simulink model "powertrain"  (R2020b)
settings: Solver=FixedStepAuto  StartTime=0.0  StopTime=t(end)  RelTol=1e-3
PreLoadFcn:
  | C_sc = 1;
StartFcn:
  | C_sc = 1;
values from neighbouring files (symbols this model uses):
  D = 0    [model_fc.m]
  Ts = old_data.Ts    [model_fc.m]
undefined symbols (not defined in the file or in its folder): ANFIS, command, DiscIntNeverNeededParam, ECMS, Flight, in, Ion, Lithium, MPC, out, Tmpc, w
libraries: powerlib x25, neural x25, fuzblock x5, electricdrivelib x3, lib_converters x3, simulink x3, re_lib x1
(part 3 of 8)

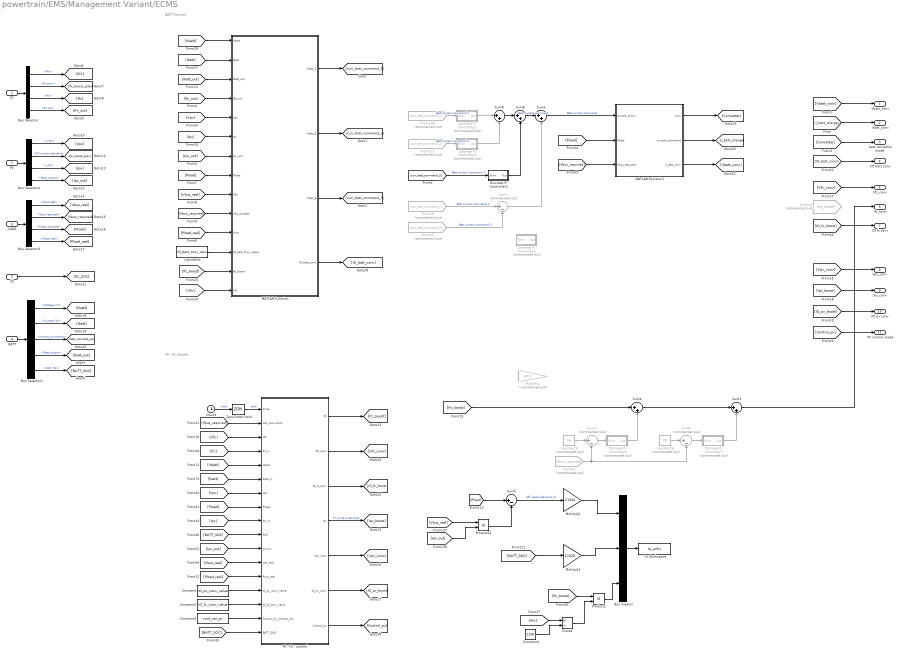
== system powertrain/EMS/Management Variant/ECMS ==
  note: PV - FC Control
  note: BATT Control
  PV : Inport
  FC : Inport  Port=2
  SC : Inport  Port=3
  BATT : Inport  Port=4
  LOAD : Inport  Port=5
  Bus Creator : BusCreator  Inputs=3
  Bus Selector : BusSelector  OutputSignals=Vfc,Ifc conv,Ifc,Ifc out
  Bus Selector1 : BusSelector  OutputSignals=Voltage (V),Current (A),current_command,Ibatt_output,SOC (%)
  Bus Selector2 : BusSelector  OutputSignals=V_PV,PV current demand,I_PV,Ibatt_output
  Bus Selector3 : BusSelector  OutputSignals=Vbus real,Vbus required,Pload required,Pload real
  Clock3 : Clock
  Constant : Constant  Value=IO_pv_conv_value
  Constant1 : Constant  Value=1100
  Constant2 : Constant  Value=IO_fc_conv_value
  Constant3 : Constant  Value=cont_var_pv
  Constant4 : Constant  Value=IO_batt_conv_value
  Constant5 : Constant  Commented=on  Value=74
  Constant6 : Constant  Commented=on  Value=70
  Discrete PI Controller1 : Subsystem  Commented=on  DialogController=POWERSYS.PowerSysDialog  mask(Discrete PI Controller){Kp=1, Ki=10, Par_Limits=[100 -100], Init=0, Ts=1e-4}
      mask prompts: Kp "Proportional gain (Kp):"; Ki "Integral gain (Ki):"; Par_Limits "Output limits: [ Upper   Lower ]"; Init "Output initial value:"; Ts "Sample time:"
      mask help: This block implements a discrete PI controller.
      mask init:
      | UpperLimit=Par_Limits(1);
      | LowerLimit=Par_Limits(2);
      | power_initmask();
      mask Help: This block is part of a subset of blocks in the Extras library that does not have documentation associated with it, other than the block mask description.
      mask Display: disp('PI');
  Discrete PI Controller2 : Subsystem  DialogController=POWERSYS.PowerSysDialog  mask(Discrete PI Controller){Kp=10, Ki=100, Par_Limits=[30 -4], Init=0, Ts=Ts}
      mask prompts: Kp "Proportional gain (Kp):"; Ki "Integral gain (Ki):"; Par_Limits "Output limits: [ Upper   Lower ]"; Init "Output initial value:"; Ts "Sample time:"
      mask help: This block implements a discrete PI controller.
      mask init:
      | UpperLimit=Par_Limits(1);
      | LowerLimit=Par_Limits(2);
      | power_initmask();
      mask Help: This block is part of a subset of blocks in the Extras library that does not have documentation associated with it, other than the block mask description.
      mask Display: disp('PI');
  Discrete PI Controller3 : Subsystem  Commented=on  DialogController=POWERSYS.PowerSysDialog  mask(Discrete PI Controller){Kp=10, Ki=1, Par_Limits=[100 -100], Init=0, Ts=1e-4}
      mask prompts: Kp "Proportional gain (Kp):"; Ki "Integral gain (Ki):"; Par_Limits "Output limits: [ Upper   Lower ]"; Init "Output initial value:"; Ts "Sample time:"
      mask help: This block implements a discrete PI controller.
      mask init:
      | UpperLimit=Par_Limits(1);
      | LowerLimit=Par_Limits(2);
      | power_initmask();
      mask Help: This block is part of a subset of blocks in the Extras library that does not have documentation associated with it, other than the block mask description.
      mask Display: disp('PI');
  Discrete PI Controller5 : Subsystem  Commented=on  DialogController=POWERSYS.PowerSysDialog  mask(Discrete PI Controller){Kp=10, Ki=10, Par_Limits=[50 -20], Init=0, Ts=1e-4}
      mask prompts: Kp "Proportional gain (Kp):"; Ki "Integral gain (Ki):"; Par_Limits "Output limits: [ Upper   Lower ]"; Init "Output initial value:"; Ts "Sample time:"
      mask help: This block implements a discrete PI controller.
      mask init:
      | UpperLimit=Par_Limits(1);
      | LowerLimit=Par_Limits(2);
      | power_initmask();
      mask Help: This block is part of a subset of blocks in the Extras library that does not have documentation associated with it, other than the block mask description.
      mask Display: disp('PI');
  Discrete PI Controller6 : Subsystem  Commented=on  DialogController=POWERSYS.PowerSysDialog  mask(Discrete PI Controller){Kp=10, Ki=10, Par_Limits=[40 0], Init=0, Ts=1e-4}
      mask prompts: Kp "Proportional gain (Kp):"; Ki "Integral gain (Ki):"; Par_Limits "Output limits: [ Upper   Lower ]"; Init "Output initial value:"; Ts "Sample time:"
      mask help: This block implements a discrete PI controller.
      mask init:
      | UpperLimit=Par_Limits(1);
      | LowerLimit=Par_Limits(2);
      | power_initmask();
      mask Help: This block is part of a subset of blocks in the Extras library that does not have documentation associated with it, other than the block mask description.
      mask Display: disp('PI');
  Discrete PI Controller7 : Subsystem  Commented=on  DialogController=POWERSYS.PowerSysDialog  mask(Discrete PI Controller){Kp=10, Ki=10, Par_Limits=[0 -40], Init=0, Ts=1e-4}
      mask prompts: Kp "Proportional gain (Kp):"; Ki "Integral gain (Ki):"; Par_Limits "Output limits: [ Upper   Lower ]"; Init "Output initial value:"; Ts "Sample time:"
      mask help: This block implements a discrete PI controller.
      mask init:
      | UpperLimit=Par_Limits(1);
      | LowerLimit=Par_Limits(2);
      | power_initmask();
      mask Help: This block is part of a subset of blocks in the Extras library that does not have documentation associated with it, other than the block mask description.
      mask Display: disp('PI');
  Divide : Product  Inputs=*/
  From108 : From  Commented=on  GotoTag=curr_batt_command_1
  From110 : From  Commented=on  GotoTag=curr_batt_command_2
  From16 : From  Commented=on  GotoTag=Ifc_boost
  From25 : From  Commented=on  GotoTag=curr_batt_command_3
  From26 : From  Commented=on  GotoTag=curr_batt_command_1
  From30 : From  Commented=on  GotoTag=Vbus_required
  MATLAB Function : MATLAB Function  TreatAsAtomicUnit=on
  MATLAB Function1 : MATLAB Function  TreatAsAtomicUnit=on
  Multiply1 : Gain  Commented=on  Gain=1/0.9
  Multiply2 : Gain  Gain=1/1500
  Multiply3 : Gain  Gain=1/100
  PV - FC - control : MATLAB Function  TreatAsAtomicUnit=on
  Product1 : Product
  Product21 : Product
  Sum1 : Sum  Commented=on  Inputs=|+-
  Sum{2..4,8..9} (5 alike) : Sum  Inputs=|++
  Sum5 : Sum  Inputs=|+-
  Sum6 : Sum  Commented=on  Inputs=|+-
  Sum7 : Sum  Commented=on  Inputs=|+-
  To Workspace : ToWorkspace  VariableName=to_anfis  SaveFormat=Timeseries  SampleTime=-1
  Zero-Order Hold : ZeroOrderHold  SampleTime=Ts
  Vbatt_conv : Outport
  Ibatt_conv : Outport  Port=2
  batt converter mode : Outport  Port=3
  I/O batt conv : Outport  Port=4
  Vfc_conv : Outport  Port=5
  Ifc_conv : Outport  Port=6
  I/O fc conv : Outport  Port=7
  Vpv_conv : Outport  Port=8
  Ipv_conv : Outport  Port=9
  I/O pv conv : Outport  Port=10
  PV control mode : Outport  Port=11
  wires:
  [Ipv_out] -> PV - FC - control/11(Ipvout)
  Sum1/1 -> Sum2/2
  PV - FC - control/7(Control_pv) -> [Control_pv]
  [Vbus_required] -> PV - FC - control/2(Vdc_command)
  MATLAB Function/4(IO_batt_conv) -> [IO_batt_conv]
  Constant3/1 -> PV - FC - control/16(Control_pv_choose_var)
  [Vbatt_conv] -> Vbatt_conv/1
  [Vbus_real] -> PV - FC - control/12(Vdc_real)
  [Pload] -> MATLAB Function/8(Pload)
  Zero-Order Hold/1 -> PV - FC - control/1(Time)  "time"
  [Ipv] -> PV - FC - control/9(Ipv_in)
  Sum8/1 -> Sum2/1  "Batt current command"
  [Vpv] -> PV - FC - control/7(Vpv)
  LOAD/1 -> Bus Selector3/1
  Clock3/1 -> Zero-Order Hold/1  "time"
  [Control_pv] -> PV control mode/1
  [Ipv_out] -> MATLAB Function/7(Ipv_out)
  Bus Selector/3 -> [Ifc]  "<Ifc>"
  [IO_batt_conv] -> I/O batt conv/1
  Bus Selector3/3 -> [Pload]  "<Pload required>"
  PV - FC - control/4(Ipv) -> [Ipv_boost]  "PV current demand"
  Bus Selector2/4 -> [Ipv_out]  "<Ibatt_output>"
  [Ifc_boost] -> Sum4/1
  [Vbus_required] -> MATLAB Function/10(Vdc_wanted)
  [BATT_SOC] -> PV - FC - control/17(BATT_SOC)
  PV/1 -> Bus Selector2/1
  [curr_batt_command_3] -> Discrete PI Controller2/1(Error)  "Batt current command 3"
  From110/1 -> Discrete PI Controller3/1(Error)  "Batt current command 3"
  [Vbus_required] -> MATLAB Function1/3(Vbus_required)
  Bus Selector1/3 -> [Ibatt_command_pre]  "<current_command>"
  PV - FC - control/3(IO_fc_conv) -> [IO_fc_boost]
  [Ifc_out] -> MATLAB Function/4(Ifc_out)
  [Vpv_conv] -> Vpv_conv/1
  Bus Selector1/2 -> [Ibatt]  "<Current (A)>"
  MATLAB Function1/3(V_batt_conv) -> [Vbatt_conv]
  [Ifc_boost] -> MATLAB Function/13(Ifc_boost)
  Bus Selector/2 -> [Ifc_boost_prev]  "<Ifc conv>"
  Bus Selector3/4 -> [Pload_real]  "<Pload real>"
  Discrete PI Controller3/1(Out) -> Sum9/2
  [Ifc] -> PV - FC - control/4(Ifc_in)
  Discrete PI Controller6/1(Out) -> Sum4/2
  [Vbatt] -> MATLAB Function/1(Vbatt)
  PV - FC - control/6(IO_pv_conv) -> [IO_pv_boost]
  Discrete PI Controller2/1(Out) -> Sum8/2
  Bus Selector1/5 -> [BATT_SOC]  "<SOC (%)>"
  Bus Selector1/4 -> [Ibatt_out]  "<Ibatt_output>"
  [Vbatt] -> PV - FC - control/5(Vbatt)
  [Ipv_boost] -> Ipv_conv/1
  Sum7/1 -> Discrete PI Controller6/1(Error)
  Bus Selector3/2 -> [Vbus_required]  "<Vbus required>"
  Bus Selector3/1 -> [Vbus_real]  "<Vbus real>"
  Bus Selector2/2 -> [Ipv_boost_prev]  "<PV current demand>"
  FC/1 -> Bus Selector/1
  PV - FC - control/2(Vfc_conv) -> [Vfc_conv]
  Bus Selector/4 -> [Ifc_out]  "<Ifc out>"
  PV - FC - control/1(Ifc) -> [Ifc_boost]
  [BATT_SOC] -> PV - FC - control/10(SOC)
  [Vfc] -> PV - FC - control/3(Vfc)
  [Pload] -> PV - FC - control/8(Pload)
  Sum6/1 -> Discrete PI Controller7/1(Error)
  From26/1 -> Sum1/1  "Batt current command 1"
  [Pload_real] -> MATLAB Function/11(Pout)
  PV - FC - control/5(Vpv_conv) -> [Vpv_conv]
  MATLAB Function1/2(current_command) -> [I_batt_charge]
  [Ibatt_out] -> MATLAB Function/3(Ibatt_out)
  Constant6/1 -> Sum6/1
  Sum4/1 -> Sum3/1
  SC/1 -> [SC_SOC]
  [Ipv] -> MATLAB Function/6(Ipv)
  Bus Selector2/1 -> [Vpv]  "<V_PV>"
  Constant2/1 -> PV - FC - control/15(IO_fc_conv_value)
  [Pload] -> MATLAB Function1/2(Pload)
  MATLAB Function/1(Ibatt_1) -> [curr_batt_command_1]
  Constant5/1 -> Sum7/1
  Constant4/1 -> MATLAB Function/12(IO_batt_conv_value)
  MATLAB Function/2(Ibatt_2) -> [curr_batt_command_2]
  [IO_fc_boost] -> I/O fc conv/1
  [Ibatt] -> MATLAB Function/2(Ibatt)
  From108/1 -> Discrete PI Controller1/1(Error)  "Batt current command 1"
  [IO_pv_boost] -> I/O pv conv/1
  Bus Selector2/3 -> [Ipv]  "<I_PV>"
  [Vfc] -> MATLAB Function/14(Vfc)
  MATLAB Function/3(Ibatt_3) -> [curr_batt_command_3]
  From25/1 -> Sum1/2  "Batt current command 3"
  BATT/1 -> Bus Selector1/1
  Sum3/1 -> Ifc_conv/1
  [Vfc_conv] -> Vfc_conv/1
  Sum2/1 -> MATLAB Function1/1(current_comm)  "Batt current command"
  Bus Selector/1 -> [Vfc]  "<Vfc>"
  [Pload_real] -> PV - FC - control/13(Pout_real)
  [Ibatt] -> PV - FC - control/6(Ibatt_in)
  [Vpv] -> MATLAB Function/5(Vpv)
  [Vbus_real] -> MATLAB Function/9(Vdc)
  Discrete PI Controller7/1(Out) -> Sum3/2
  Bus Selector1/1 -> [Vbatt]  "<Voltage (V)>"
  Sum9/1 -> Sum8/1
  [Converter] -> batt converter mode/1
  MATLAB Function1/1(conv) -> [Converter]
  Constant/1 -> PV - FC - control/14(IO_pv_conv_value)
  [I_batt_charge] -> Ibatt_conv/1
  From30/1 -> Sum6/2, Sum7/2
  Discrete PI Controller1/1(Out) -> Sum9/1
  [Vbus_real] -> Product21/1
  [Ipv_out] -> Product21/2
  [BATT_SOC] -> Multiply3/1
  [Pload] -> Sum5/1
  Sum5/1 -> Multiply2/1  "diff pload pdemand_fc"
  Multiply3/1 -> Bus Creator/2
  Product21/1 -> Sum5/2
  Multiply2/1 -> Bus Creator/1
  [Ifc_boost] -> Product1/1
  Divide/1 -> Product1/2
  Product1/1 -> Bus Creator/3
  Bus Creator/1 -> To Workspace/1
  Constant1/1 -> Divide/2
  [Vfc] -> Divide/1

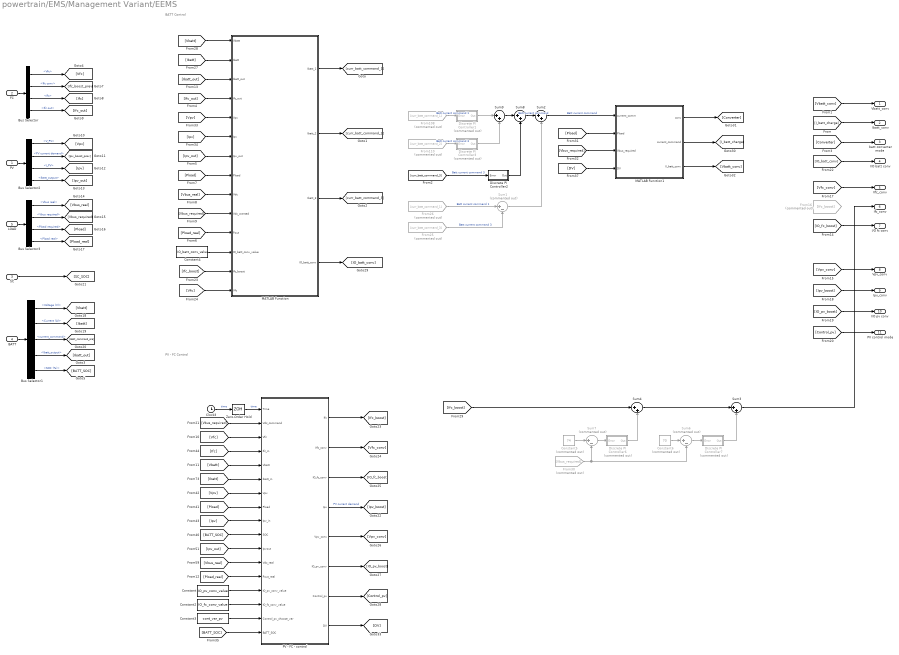
== system powertrain/EMS/Management Variant/EEMS ==
  note: PV - FC Control
  note: BATT Control
  PV : Inport
  FC : Inport  Port=2
  SC : Inport  Port=3
  BATT : Inport  Port=4
  LOAD : Inport  Port=5
  Bus Selector : BusSelector  OutputSignals=Vfc,Ifc conv,Ifc,Ifc out
  Bus Selector1 : BusSelector  OutputSignals=Voltage (V),Current (A),current_command,Ibatt_output,SOC (%)
  Bus Selector2 : BusSelector  OutputSignals=V_PV,PV current demand,I_PV,Ibatt_output
  Bus Selector3 : BusSelector  OutputSignals=Vbus real,Vbus required,Pload required,Pload real
  Clock3 : Clock
  Constant : Constant  Value=IO_pv_conv_value
  Constant2 : Constant  Value=IO_fc_conv_value
  Constant3 : Constant  Value=cont_var_pv
  Constant4 : Constant  Value=IO_batt_conv_value
  Constant5 : Constant  Commented=on  Value=74
  Constant6 : Constant  Commented=on  Value=70
  Discrete PI Controller1 : Subsystem  Commented=on  DialogController=POWERSYS.PowerSysDialog  mask(Discrete PI Controller){Kp=1, Ki=10, Par_Limits=[100 -100], Init=0, Ts=1e-4}
      mask prompts: Kp "Proportional gain (Kp):"; Ki "Integral gain (Ki):"; Par_Limits "Output limits: [ Upper   Lower ]"; Init "Output initial value:"; Ts "Sample time:"
      mask help: This block implements a discrete PI controller.
      mask init:
      | UpperLimit=Par_Limits(1);
      | LowerLimit=Par_Limits(2);
      | power_initmask();
      mask Help: This block is part of a subset of blocks in the Extras library that does not have documentation associated with it, other than the block mask description.
      mask Display: disp('PI');
  Discrete PI Controller2 : Subsystem  DialogController=POWERSYS.PowerSysDialog  mask(Discrete PI Controller){Kp=10, Ki=100, Par_Limits=[30 -4], Init=0, Ts=Ts}
      mask prompts: Kp "Proportional gain (Kp):"; Ki "Integral gain (Ki):"; Par_Limits "Output limits: [ Upper   Lower ]"; Init "Output initial value:"; Ts "Sample time:"
      mask help: This block implements a discrete PI controller.
      mask init:
      | UpperLimit=Par_Limits(1);
      | LowerLimit=Par_Limits(2);
      | power_initmask();
      mask Help: This block is part of a subset of blocks in the Extras library that does not have documentation associated with it, other than the block mask description.
      mask Display: disp('PI');
  Discrete PI Controller3 : Subsystem  Commented=on  DialogController=POWERSYS.PowerSysDialog  mask(Discrete PI Controller){Kp=10, Ki=1, Par_Limits=[100 -100], Init=0, Ts=1e-4}
      mask prompts: Kp "Proportional gain (Kp):"; Ki "Integral gain (Ki):"; Par_Limits "Output limits: [ Upper   Lower ]"; Init "Output initial value:"; Ts "Sample time:"
      mask help: This block implements a discrete PI controller.
      mask init:
      | UpperLimit=Par_Limits(1);
      | LowerLimit=Par_Limits(2);
      | power_initmask();
      mask Help: This block is part of a subset of blocks in the Extras library that does not have documentation associated with it, other than the block mask description.
      mask Display: disp('PI');
  Discrete PI Controller6 : Subsystem  Commented=on  DialogController=POWERSYS.PowerSysDialog  mask(Discrete PI Controller){Kp=10, Ki=10, Par_Limits=[40 0], Init=0, Ts=1e-4}
      mask prompts: Kp "Proportional gain (Kp):"; Ki "Integral gain (Ki):"; Par_Limits "Output limits: [ Upper   Lower ]"; Init "Output initial value:"; Ts "Sample time:"
      mask help: This block implements a discrete PI controller.
      mask init:
      | UpperLimit=Par_Limits(1);
      | LowerLimit=Par_Limits(2);
      | power_initmask();
      mask Help: This block is part of a subset of blocks in the Extras library that does not have documentation associated with it, other than the block mask description.
      mask Display: disp('PI');
  Discrete PI Controller7 : Subsystem  Commented=on  DialogController=POWERSYS.PowerSysDialog  mask(Discrete PI Controller){Kp=10, Ki=10, Par_Limits=[0 -40], Init=0, Ts=1e-4}
      mask prompts: Kp "Proportional gain (Kp):"; Ki "Integral gain (Ki):"; Par_Limits "Output limits: [ Upper   Lower ]"; Init "Output initial value:"; Ts "Sample time:"
      mask help: This block implements a discrete PI controller.
      mask init:
      | UpperLimit=Par_Limits(1);
      | LowerLimit=Par_Limits(2);
      | power_initmask();
      mask Help: This block is part of a subset of blocks in the Extras library that does not have documentation associated with it, other than the block mask description.
      mask Display: disp('PI');
  From108 : From  Commented=on  GotoTag=curr_batt_command_1
  From110 : From  Commented=on  GotoTag=curr_batt_command_2
  From16 : From  Commented=on  GotoTag=Ifc_boost
  From25 : From  Commented=on  GotoTag=curr_batt_command_3
  From26 : From  Commented=on  GotoTag=curr_batt_command_1
  From30 : From  Commented=on  GotoTag=Vbus_required
  MATLAB Function : MATLAB Function  TreatAsAtomicUnit=on
  MATLAB Function1 : MATLAB Function  TreatAsAtomicUnit=on
  PV - FC - control : MATLAB Function  TreatAsAtomicUnit=on
  Sum1 : Sum  Commented=on  Inputs=|+-
  Sum{2..4,8..9} (5 alike) : Sum  Inputs=|++
  Sum6 : Sum  Commented=on  Inputs=|+-
  Sum7 : Sum  Commented=on  Inputs=|+-
  Zero-Order Hold : ZeroOrderHold  SampleTime=Ts
  Vbatt_conv : Outport
  Ibatt_conv : Outport  Port=2
  batt converter mode : Outport  Port=3
  I/O batt conv : Outport  Port=4
  Vfc_conv : Outport  Port=5
  Ifc_conv : Outport  Port=6
  I/O fc conv : Outport  Port=7
  Vpv_conv : Outport  Port=8
  Ipv_conv : Outport  Port=9
  I/O pv conv : Outport  Port=10
  PV control mode : Outport  Port=11
  wires:
  [Ipv_out] -> PV - FC - control/11(Ipvout)
  Sum1/1 -> Sum2/2
  PV - FC - control/7(Control_pv) -> [Control_pv]
  [Vbus_required] -> PV - FC - control/2(Vdc_command)
  MATLAB Function/4(IO_batt_conv) -> [IO_batt_conv]
  Constant3/1 -> PV - FC - control/16(Control_pv_choose_var)
  [Vbatt_conv] -> Vbatt_conv/1
  [Vbus_real] -> PV - FC - control/12(Vdc_real)
  [Pload] -> MATLAB Function/8(Pload)
  Zero-Order Hold/1 -> PV - FC - control/1(Time)  "time"
  [Ipv] -> PV - FC - control/9(Ipv_in)
  Sum8/1 -> Sum2/1  "Batt current command"
  [Vpv] -> PV - FC - control/7(Vpv)
  LOAD/1 -> Bus Selector3/1
  Clock3/1 -> Zero-Order Hold/1  "time"
  [Control_pv] -> PV control mode/1
  [Ipv_out] -> MATLAB Function/7(Ipv_out)
  Bus Selector/3 -> [Ifc]  "<Ifc>"
  [IO_batt_conv] -> I/O batt conv/1
  Bus Selector3/3 -> [Pload]  "<Pload required>"
  PV - FC - control/4(Ipv) -> [Ipv_boost]  "PV current demand"
  Bus Selector2/4 -> [Ipv_out]  "<Ibatt_output>"
  [Ifc_boost] -> Sum4/1
  [Vbus_required] -> MATLAB Function/10(Vdc_wanted)
  [BATT_SOC] -> PV - FC - control/17(BATT_SOC)
  PV/1 -> Bus Selector2/1
  [curr_batt_command_3] -> Discrete PI Controller2/1(Error)  "Batt current command 3"
  From110/1 -> Discrete PI Controller3/1(Error)  "Batt current command 3"
  [Vbus_required] -> MATLAB Function1/3(Vbus_required)
  Bus Selector1/3 -> [Ibatt_command_pre]  "<current_command>"
  PV - FC - control/3(IO_fc_conv) -> [IO_fc_boost]
  [Ifc_out] -> MATLAB Function/4(Ifc_out)
  [Vpv_conv] -> Vpv_conv/1
  Bus Selector1/2 -> [Ibatt]  "<Current (A)>"
  MATLAB Function1/3(V_batt_conv) -> [Vbatt_conv]
  [Ifc_boost] -> MATLAB Function/13(Ifc_boost)
  Bus Selector/2 -> [Ifc_boost_prev]  "<Ifc conv>"
  Bus Selector3/4 -> [Pload_real]  "<Pload real>"
  Discrete PI Controller3/1(Out) -> Sum9/2
  [Ifc] -> PV - FC - control/4(Ifc_in)
  Discrete PI Controller6/1(Out) -> Sum4/2
  [Vbatt] -> MATLAB Function/1(Vbatt)
  PV - FC - control/6(IO_pv_conv) -> [IO_pv_boost]
  Discrete PI Controller2/1(Out) -> Sum8/2
  Bus Selector1/5 -> [BATT_SOC]  "<SOC (%)>"
  Bus Selector1/4 -> [Ibatt_out]  "<Ibatt_output>"
  [Vbatt] -> PV - FC - control/5(Vbatt)
  [Ipv_boost] -> Ipv_conv/1
  Sum7/1 -> Discrete PI Controller6/1(Error)
  Bus Selector3/2 -> [Vbus_required]  "<Vbus required>"
  Bus Selector3/1 -> [Vbus_real]  "<Vbus real>"
  Bus Selector2/2 -> [Ipv_boost_prev]  "<PV current demand>"
  FC/1 -> Bus Selector/1
  PV - FC - control/2(Vfc_conv) -> [Vfc_conv]
  Bus Selector/4 -> [Ifc_out]  "<Ifc out>"
  PV - FC - control/1(Ifc) -> [Ifc_boost]
  [BATT_SOC] -> PV - FC - control/10(SOC)
  [Vfc] -> PV - FC - control/3(Vfc)
  [Pload] -> PV - FC - control/8(Pload)
  Sum6/1 -> Discrete PI Controller7/1(Error)
  From26/1 -> Sum1/1  "Batt current command 1"
  [Pload_real] -> MATLAB Function/11(Pout)
  PV - FC - control/5(Vpv_conv) -> [Vpv_conv]
  MATLAB Function1/2(current_command) -> [I_batt_charge]
  [Ibatt_out] -> MATLAB Function/3(Ibatt_out)
  Constant6/1 -> Sum6/1
  Sum4/1 -> Sum3/1
  SC/1 -> [SC_SOC]
  [Ipv] -> MATLAB Function/6(Ipv)
  Bus Selector2/1 -> [Vpv]  "<V_PV>"
  Constant2/1 -> PV - FC - control/15(IO_fc_conv_value)
  [Pload] -> MATLAB Function1/2(Pload)
  MATLAB Function/1(Ibatt_1) -> [curr_batt_command_1]
  Constant5/1 -> Sum7/1
  Constant4/1 -> MATLAB Function/12(IO_batt_conv_value)
  MATLAB Function/2(Ibatt_2) -> [curr_batt_command_2]
  [IO_fc_boost] -> I/O fc conv/1
  [Ibatt] -> MATLAB Function/2(Ibatt)
  From108/1 -> Discrete PI Controller1/1(Error)  "Batt current command 1"
  [IO_pv_boost] -> I/O pv conv/1
  Bus Selector2/3 -> [Ipv]  "<I_PV>"
  [Vfc] -> MATLAB Function/14(Vfc)
  MATLAB Function/3(Ibatt_3) -> [curr_batt_command_3]
  From25/1 -> Sum1/2  "Batt current command 3"
  BATT/1 -> Bus Selector1/1
  Sum3/1 -> Ifc_conv/1
  [Vfc_conv] -> Vfc_conv/1
  Sum2/1 -> MATLAB Function1/1(current_comm)  "Batt current command"
  Bus Selector/1 -> [Vfc]  "<Vfc>"
  [Pload_real] -> PV - FC - control/13(Pout_real)
  [Ibatt] -> PV - FC - control/6(Ibatt_in)
  [Vpv] -> MATLAB Function/5(Vpv)
  [Vbus_real] -> MATLAB Function/9(Vdc)
  Discrete PI Controller7/1(Out) -> Sum3/2
  Bus Selector1/1 -> [Vbatt]  "<Voltage (V)>"
  Sum9/1 -> Sum8/1
  [Converter] -> batt converter mode/1
  MATLAB Function1/1(conv) -> [Converter]
  Constant/1 -> PV - FC - control/14(IO_pv_conv_value)
  [I_batt_charge] -> Ibatt_conv/1
  From30/1 -> Sum6/2, Sum7/2
  Discrete PI Controller1/1(Out) -> Sum9/1
  PV - FC - control/8(DV) -> [DV]
  [DV] -> MATLAB Function1/4(DV)

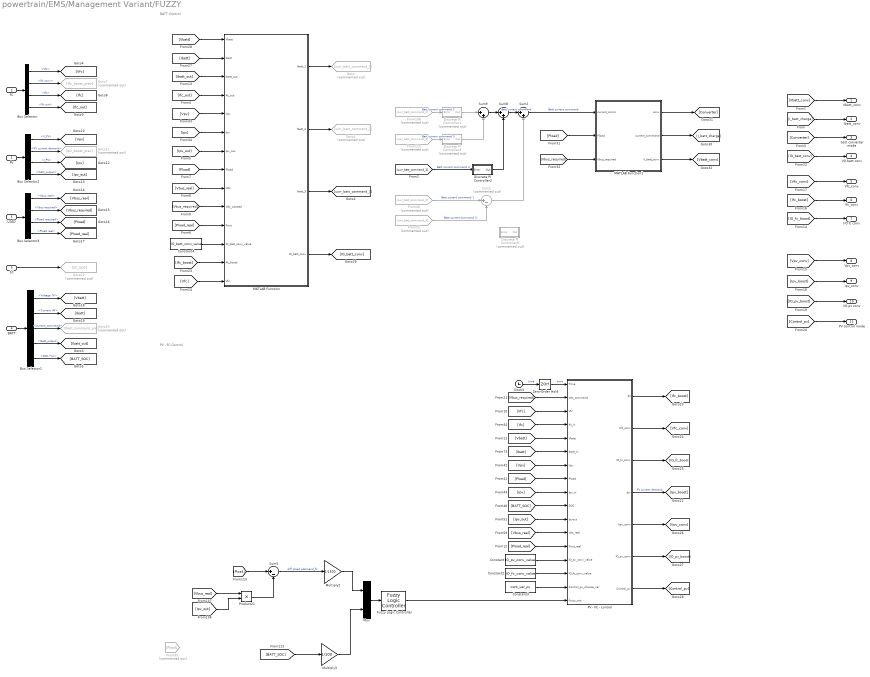
== system powertrain/EMS/Management Variant/FUZZY ==
  note: BATT Control
  note: PV - FC Control
  PV : Inport
  FC : Inport  Port=2
  SC : Inport  Port=3
  BATT : Inport  Port=4
  LOAD : Inport  Port=5
  Bus Selector : BusSelector  OutputSignals=Vfc,Ifc conv,Ifc,Ifc out
  Bus Selector1 : BusSelector  OutputSignals=Voltage (V),Current (A),current_command,Ibatt_output,SOC (%)
  Bus Selector2 : BusSelector  OutputSignals=V_PV,PV current demand,I_PV,Ibatt_output
  Bus Selector3 : BusSelector  OutputSignals=Vbus real,Vbus required,Pload required,Pload real
  Clock3 : Clock
  Constant : Constant  Value=IO_pv_conv_value
  Constant2 : Constant  Value=IO_fc_conv_value
  Constant3 : Constant  Value=cont_var_pv
  Constant4 : Constant  Value=IO_batt_conv_value
  Discrete PI Controller1 : Subsystem  Commented=on  DialogController=POWERSYS.PowerSysDialog  mask(Discrete PI Controller){Kp=1, Ki=10, Par_Limits=[100 -100], Init=0, Ts=1e-4}
      mask prompts: Kp "Proportional gain (Kp):"; Ki "Integral gain (Ki):"; Par_Limits "Output limits: [ Upper   Lower ]"; Init "Output initial value:"; Ts "Sample time:"
      mask help: This block implements a discrete PI controller.
      mask init:
      | UpperLimit=Par_Limits(1);
      | LowerLimit=Par_Limits(2);
      | power_initmask();
      mask Help: This block is part of a subset of blocks in the Extras library that does not have documentation associated with it, other than the block mask description.
      mask Display: disp('PI');
  Discrete PI Controller2 : Subsystem  DialogController=POWERSYS.PowerSysDialog  mask(Discrete PI Controller){Kp=10, Ki=100, Par_Limits=[30 -4], Init=0, Ts=Ts}
      mask prompts: Kp "Proportional gain (Kp):"; Ki "Integral gain (Ki):"; Par_Limits "Output limits: [ Upper   Lower ]"; Init "Output initial value:"; Ts "Sample time:"
      mask help: This block implements a discrete PI controller.
      mask init:
      | UpperLimit=Par_Limits(1);
      | LowerLimit=Par_Limits(2);
      | power_initmask();
      mask Help: This block is part of a subset of blocks in the Extras library that does not have documentation associated with it, other than the block mask description.
      mask Display: disp('PI');
  Discrete PI Controller3 : Subsystem  Commented=on  DialogController=POWERSYS.PowerSysDialog  mask(Discrete PI Controller){Kp=10, Ki=1, Par_Limits=[100 -100], Init=0, Ts=1e-4}
      mask prompts: Kp "Proportional gain (Kp):"; Ki "Integral gain (Ki):"; Par_Limits "Output limits: [ Upper   Lower ]"; Init "Output initial value:"; Ts "Sample time:"
      mask help: This block implements a discrete PI controller.
      mask init:
      | UpperLimit=Par_Limits(1);
      | LowerLimit=Par_Limits(2);
      | power_initmask();
      mask Help: This block is part of a subset of blocks in the Extras library that does not have documentation associated with it, other than the block mask description.
      mask Display: disp('PI');
  Discrete PI Controller5 : Subsystem  Commented=on  DialogController=POWERSYS.PowerSysDialog  mask(Discrete PI Controller){Kp=10, Ki=10, Par_Limits=[50 -20], Init=0, Ts=1e-4}
      mask prompts: Kp "Proportional gain (Kp):"; Ki "Integral gain (Ki):"; Par_Limits "Output limits: [ Upper   Lower ]"; Init "Output initial value:"; Ts "Sample time:"
      mask help: This block implements a discrete PI controller.
      mask init:
      | UpperLimit=Par_Limits(1);
      | LowerLimit=Par_Limits(2);
      | power_initmask();
      mask Help: This block is part of a subset of blocks in the Extras library that does not have documentation associated with it, other than the block mask description.
      mask Display: disp('PI');
  From108 : From  Commented=on  GotoTag=curr_batt_command_1
  From110 : From  Commented=on  GotoTag=curr_batt_command_2
  From25 : From  Commented=on  GotoTag=curr_batt_command_3
  From26 : From  Commented=on  GotoTag=curr_batt_command_1
  From35 : From  Commented=on  GotoTag=Pload
  Fuzzy Logic Controller : fuzblock/Fuzzy Logic  Controller  FIS='test_fis_paper.fis'  OutputSampleNumber=10  DataType=double  FuzzifiedInputs=off  RuleFiringStrengths=off  RuleOutputs=off  AggregatedOutputs=off  SimulateUsing=Code generation  OutOfRangeInputValueMessage=warning  NoRuleFiredMessage=warning  EmptyOutputFuzzySetMessage=warning
  Goto : Goto  Commented=on  GotoTag=curr_batt_command_1
  Goto1 : Goto  Commented=on  GotoTag=curr_batt_command_2
  Goto11 : Goto  Commented=on  GotoTag=Ipv_boost_prev
  Goto20 : Goto  Commented=on  GotoTag=Ibatt_command_pre
  Goto21 : Goto  Commented=on  GotoTag=SC_SOC
  Goto7 : Goto  Commented=on  GotoTag=Ifc_boost_prev
  MATLAB Function : MATLAB Function  TreatAsAtomicUnit=on
  MATLAB Function1 : MATLAB Function  TreatAsAtomicUnit=on
  Multiply2 : Gain  Gain=1/1500
  Multiply3 : Gain  Gain=1/100
  Mux : Mux  Inputs=2
  PV - FC - control : MATLAB Function  TreatAsAtomicUnit=on
  Product21 : Product
  Sum1 : Sum  Commented=on  Inputs=|+-
  Sum2 : Sum  Inputs=|++
  Sum5 : Sum  Inputs=|+-
  Sum8 : Sum  Inputs=|++
  Sum9 : Sum  Inputs=|++
  Zero-Order Hold : ZeroOrderHold  SampleTime=Ts
  Vbatt_conv : Outport
  Ibatt_conv : Outport  Port=2
  batt converter mode : Outport  Port=3
  I/O batt conv : Outport  Port=4
  Vfc_conv : Outport  Port=5
  Ifc_conv : Outport  Port=6
  I/O fc conv : Outport  Port=7
  Vpv_conv : Outport  Port=8
  Ipv_conv : Outport  Port=9
  I/O pv conv : Outport  Port=10
  PV control mode : Outport  Port=11
  wires:
  [Vbus_real] -> Product21/1
  Mux/1 -> Fuzzy Logic Controller/1
  Multiply3/1 -> Mux/2
  [Ipv_out] -> Product21/2
  [Pload] -> Sum5/1
  Product21/1 -> Sum5/2
  [BATT_SOC] -> Multiply3/1
  Multiply2/1 -> Mux/1
  Sum5/1 -> Multiply2/1  "diff pload pdemand_fc"
  Constant/1 -> PV - FC - control/14(IO_pv_conv_value)
  MATLAB Function1/1(conv) -> [Converter]
  [Vbatt] -> MATLAB Function/1(Vbatt)
  [Ibatt_out] -> MATLAB Function/3(Ibatt_out)
  Bus Selector1/5 -> [BATT_SOC]  "<SOC (%)>"
  [Vpv] -> MATLAB Function/5(Vpv)
  PV - FC - control/3(IO_fc_conv) -> [IO_fc_boost]
  [Ifc_out] -> MATLAB Function/4(Ifc_out)
  Bus Selector1/3 -> Goto20/1  "<current_command>"
  [IO_fc_boost] -> I/O fc conv/1
  MATLAB Function1/3(V_batt_conv) -> [Vbatt_conv]
  Bus Selector1/2 -> [Ibatt]  "<Current (A)>"
  [Ifc_boost] -> MATLAB Function/13(Ifc_boost)
  [Vbus_required] -> MATLAB Function1/3(Vbus_required)
  Sum2/1 -> MATLAB Function1/1(current_comm)  "Batt current command"
  [Vpv_conv] -> Vpv_conv/1
  Bus Selector1/1 -> [Vbatt]  "<Voltage (V)>"
  [Ibatt] -> PV - FC - control/6(Ibatt_in)
  From26/1 -> Sum1/1  "Batt current command 1"
  Bus Selector1/4 -> [Ibatt_out]  "<Ibatt_output>"
  MATLAB Function1/2(current_command) -> [I_batt_charge]
  [Ipv_boost] -> Ipv_conv/1
  [Pload_real] -> MATLAB Function/11(Pout)
  PV - FC - control/5(Vpv_conv) -> [Vpv_conv]
  Constant2/1 -> PV - FC - control/15(IO_fc_conv_value)
  MATLAB Function/2(Ibatt_2) -> Goto1/1
  MATLAB Function/1(Ibatt_1) -> Goto/1
  Bus Selector2/1 -> [Vpv]  "<V_PV>"
  [Pload] -> MATLAB Function1/2(Pload)
  From25/1 -> Sum1/2  "Batt current command 3"
  [Ibatt] -> MATLAB Function/2(Ibatt)
  [IO_pv_boost] -> I/O pv conv/1
  [Vfc] -> MATLAB Function/14(Vfc)
  Bus Selector2/3 -> [Ipv]  "<I_PV>"
  Sum1/1 -> Sum2/2
  [Vfc_conv] -> Vfc_conv/1
  [Ipv_out] -> PV - FC - control/11(Ipvout)
  PV - FC - control/7(Control_pv) -> [Control_pv]
  [Vbus_required] -> PV - FC - control/2(Vdc_command)
  [Vbatt_conv] -> Vbatt_conv/1
  [Vbus_real] -> PV - FC - control/12(Vdc_real)
  MATLAB Function/4(IO_batt_conv) -> [IO_batt_conv]
  Constant3/1 -> PV - FC - control/16(Control_pv_choose_var)
  PV - FC - control/1(Ifc) -> [Ifc_boost]
  FC/1 -> Bus Selector/1
  [Ipv] -> PV - FC - control/9(Ipv_in)
  Sum8/1 -> Sum2/1  "Batt current command"
  Zero-Order Hold/1 -> PV - FC - control/1(Time)  "time"
  [Pload] -> MATLAB Function/8(Pload)
  [Vbus_required] -> MATLAB Function/10(Vdc_wanted)
  Clock3/1 -> Zero-Order Hold/1  "time"
  [Pload_real] -> PV - FC - control/13(Pout_real)
  [Vpv] -> PV - FC - control/7(Vpv)
  LOAD/1 -> Bus Selector3/1
  [Control_pv] -> PV control mode/1
  Bus Selector/3 -> [Ifc]  "<Ifc>"
  [Ipv_out] -> MATLAB Function/7(Ipv_out)
  From110/1 -> Discrete PI Controller3/1(Error)  "Batt current command 3"
  [IO_batt_conv] -> I/O batt conv/1
  [Vbus_real] -> MATLAB Function/9(Vdc)
  Bus Selector3/3 -> [Pload]  "<Pload required>"
  Bus Selector2/4 -> [Ipv_out]  "<Ibatt_output>"
  PV - FC - control/4(Ipv) -> [Ipv_boost]  "PV current demand"
  [Ifc] -> PV - FC - control/4(Ifc_in)
  Bus Selector3/2 -> [Vbus_required]  "<Vbus required>"
  BATT/1 -> Bus Selector1/1
  Bus Selector2/2 -> Goto11/1  "<PV current demand>"
  Bus Selector3/1 -> [Vbus_real]  "<Vbus real>"
  Constant4/1 -> MATLAB Function/12(IO_batt_conv_value)
  PV - FC - control/6(IO_pv_conv) -> [IO_pv_boost]
  SC/1 -> Goto21/1
  [Converter] -> batt converter mode/1
  PV - FC - control/2(Vfc_conv) -> [Vfc_conv]
  [I_batt_charge] -> Ibatt_conv/1
  [Vbatt] -> PV - FC - control/5(Vbatt)
  [Vfc] -> PV - FC - control/3(Vfc)
  [curr_batt_command_3] -> Discrete PI Controller2/1(Error)  "Batt current command 3"
  Bus Selector/1 -> [Vfc]  "<Vfc>"
  Bus Selector/4 -> [Ifc_out]  "<Ifc out>"
  PV/1 -> Bus Selector2/1
  [Pload] -> PV - FC - control/8(Pload)
  Bus Selector/2 -> Goto7/1  "<Ifc conv>"
  Sum9/1 -> Sum8/1
  From108/1 -> Discrete PI Controller1/1(Error)  "Batt current command 1"
  Discrete PI Controller2/1(Out) -> Sum8/2
  MATLAB Function/3(Ibatt_3) -> [curr_batt_command_3]
  Discrete PI Controller1/1(Out) -> Sum9/1
  Discrete PI Controller3/1(Out) -> Sum9/2
  [BATT_SOC] -> PV - FC - control/10(SOC)
  [Ipv] -> MATLAB Function/6(Ipv)
  Bus Selector3/4 -> [Pload_real]  "<Pload real>"
  [Ifc_boost] -> Ifc_conv/1
  Fuzzy Logic Controller/1 -> PV - FC - control/17(fuzzy_out)

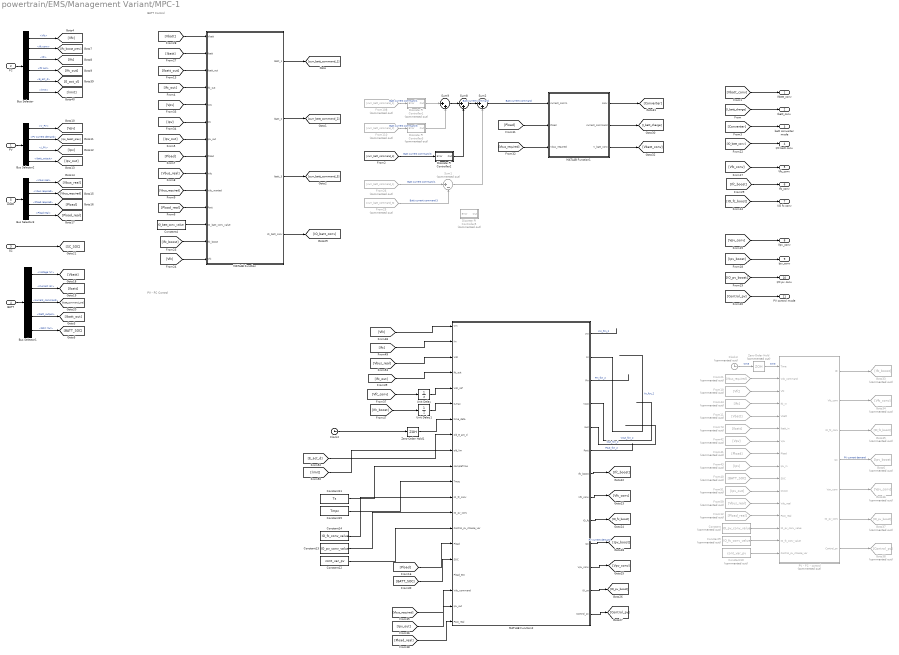
== system powertrain/EMS/Management Variant/MPC-1 ==
  note: PV - FC Control
  note: BATT Control
  PV : Inport
  FC : Inport  Port=2
  SC : Inport  Port=3
  BATT : Inport  Port=4
  LOAD : Inport  Port=5
  Bus Selector : BusSelector  OutputSignals=Vfc,Ifc conv,Ifc,Ifc out,E_act_d,limit
  Bus Selector1 : BusSelector  OutputSignals=Voltage (V),Current (A),current_command,Ibatt_output,SOC (%)
  Bus Selector2 : BusSelector  OutputSignals=V_PV,PV current demand,I_PV,Ibatt_output
  Bus Selector3 : BusSelector  OutputSignals=Vbus real,Vbus required,Pload required,Pload real
  Clock2 : Clock
  Clock3 : Clock  Commented=on
  Constant : Constant  Commented=on  Value=IO_pv_conv_value
  Constant10 : Constant  Commented=on  Value=cont_var_pv
  Constant11 : Constant  Value=Ts
  Constant12 : Constant  Value=cont_var_pv
  Constant13 : Constant  Value=IO_pv_conv_value
  Constant14 : Constant  Value=IO_fc_conv_value
  Constant15 : Constant  Value=Tmpc
  Constant4 : Constant  Value=IO_batt_conv_value
  Constant9 : Constant  Commented=on  Value=IO_fc_conv_value
  Discrete PI Controller1 : Subsystem  Commented=on  DialogController=POWERSYS.PowerSysDialog  mask(Discrete PI Controller){Kp=1, Ki=10, Par_Limits=[100 -100], Init=0, Ts=1e-4}
      mask prompts: Kp "Proportional gain (Kp):"; Ki "Integral gain (Ki):"; Par_Limits "Output limits: [ Upper   Lower ]"; Init "Output initial value:"; Ts "Sample time:"
      mask help: This block implements a discrete PI controller.
      mask init:
      | UpperLimit=Par_Limits(1);
      | LowerLimit=Par_Limits(2);
      | power_initmask();
      mask Help: This block is part of a subset of blocks in the Extras library that does not have documentation associated with it, other than the block mask description.
      mask Display: disp('PI');
  Discrete PI Controller2 : Subsystem  DialogController=POWERSYS.PowerSysDialog  mask(Discrete PI Controller){Kp=10, Ki=100, Par_Limits=[30 -4], Init=0, Ts=Ts}
      mask prompts: Kp "Proportional gain (Kp):"; Ki "Integral gain (Ki):"; Par_Limits "Output limits: [ Upper   Lower ]"; Init "Output initial value:"; Ts "Sample time:"
      mask help: This block implements a discrete PI controller.
      mask init:
      | UpperLimit=Par_Limits(1);
      | LowerLimit=Par_Limits(2);
      | power_initmask();
      mask Help: This block is part of a subset of blocks in the Extras library that does not have documentation associated with it, other than the block mask description.
      mask Display: disp('PI');
  Discrete PI Controller3 : Subsystem  Commented=on  DialogController=POWERSYS.PowerSysDialog  mask(Discrete PI Controller){Kp=10, Ki=1, Par_Limits=[100 -100], Init=0, Ts=1e-4}
      mask prompts: Kp "Proportional gain (Kp):"; Ki "Integral gain (Ki):"; Par_Limits "Output limits: [ Upper   Lower ]"; Init "Output initial value:"; Ts "Sample time:"
      mask help: This block implements a discrete PI controller.
      mask init:
      | UpperLimit=Par_Limits(1);
      | LowerLimit=Par_Limits(2);
      | power_initmask();
      mask Help: This block is part of a subset of blocks in the Extras library that does not have documentation associated with it, other than the block mask description.
      mask Display: disp('PI');
  Discrete PI Controller5 : Subsystem  Commented=on  DialogController=POWERSYS.PowerSysDialog  mask(Discrete PI Controller){Kp=10, Ki=10, Par_Limits=[50 -20], Init=0, Ts=1e-4}
      mask prompts: Kp "Proportional gain (Kp):"; Ki "Integral gain (Ki):"; Par_Limits "Output limits: [ Upper   Lower ]"; Init "Output initial value:"; Ts "Sample time:"
      mask help: This block implements a discrete PI controller.
      mask init:
      | UpperLimit=Par_Limits(1);
      | LowerLimit=Par_Limits(2);
      | power_initmask();
      mask Help: This block is part of a subset of blocks in the Extras library that does not have documentation associated with it, other than the block mask description.
      mask Display: disp('PI');
  From10 : From  Commented=on  GotoTag=Vfc
  From108 : From  Commented=on  GotoTag=curr_batt_command_1
  From11 : From  Commented=on  GotoTag=Vbatt
  From110 : From  Commented=on  GotoTag=curr_batt_command_2
  From12 : From  Commented=on  GotoTag=Pload_real
  From21 : From  Commented=on  GotoTag=Vbus_required
  From25 : From  Commented=on  GotoTag=curr_batt_command_3
  From26 : From  Commented=on  GotoTag=curr_batt_command_1
  From40 : From  Commented=on  GotoTag=BATT_SOC
  From41 : From  Commented=on  GotoTag=Pload
  From42 : From  Commented=on  GotoTag=Vpv
  From43 : From  Commented=on  GotoTag=Ipv
  From44 : From  Commented=on  GotoTag=Ifc
  From51 : From  Commented=on  GotoTag=Ipv_out
  From59 : From  Commented=on  GotoTag=Vbus_real
  From73 : From  Commented=on  GotoTag=Ibatt
  Goto33 : Goto  Commented=on  GotoTag=Ifc_boost
  Goto34 : Goto  Commented=on  GotoTag=Vfc_conv
  Goto35 : Goto  Commented=on  GotoTag=IO_fc_boost
  Goto36 : Goto  Commented=on  GotoTag=Vpv_conv
  Goto37 : Goto  Commented=on  GotoTag=IO_pv_boost
  Goto38 : Goto  Commented=on  GotoTag=Control_pv
  Goto6 : Goto  Commented=on  GotoTag=Ipv_boost
  MATLAB Function : MATLAB Function  TreatAsAtomicUnit=on
  MATLAB Function1 : MATLAB Function  TreatAsAtomicUnit=on
  MATLAB Function2 : MATLAB Function  TreatAsAtomicUnit=on
  PV - FC - control : MATLAB Function  Commented=on  TreatAsAtomicUnit=on
  Sum1 : Sum  Commented=on  Inputs=|+-
  Sum2 : Sum  Inputs=|++
  Sum8 : Sum  Inputs=|++
  Sum9 : Sum  Inputs=|++
  Unit Delay : UnitDelay  SampleTime=-1  HasFrameUpgradeWarning=on
  Unit Delay1 : UnitDelay  SampleTime=-1  HasFrameUpgradeWarning=on
  Zero-Order Hold : ZeroOrderHold  Commented=on  SampleTime=1e-4
  Zero-Order Hold1 : ZeroOrderHold  SampleTime=Ts
  Vbatt_conv : Outport
  Ibatt_conv : Outport  Port=2
  batt converter mode : Outport  Port=3
  I/O batt conv : Outport  Port=4
  Vfc_conv : Outport  Port=5
  Ifc_conv : Outport  Port=6
  I/O fc conv : Outport  Port=7
  Vpv_conv : Outport  Port=8
  Ipv_conv : Outport  Port=9
  I/O pv conv : Outport  Port=10
  PV control mode : Outport  Port=11
  wires:
  Sum1/1 -> Sum2/2
  MATLAB Function/4(IO_batt_conv) -> [IO_batt_conv]
  [Vbatt_conv] -> Vbatt_conv/1
  [Pload] -> MATLAB Function/8(Pload)
  Sum8/1 -> Sum2/1  "Batt current command"
  LOAD/1 -> Bus Selector3/1
  [Control_pv] -> PV control mode/1
  [Ipv_out] -> MATLAB Function/7(Ipv_out)
  Bus Selector/3 -> [Ifc]  "<Ifc>"
  [IO_batt_conv] -> I/O batt conv/1
  Bus Selector3/3 -> [Pload]  "<Pload required>"
  Bus Selector2/4 -> [Ipv_out]  "<Ibatt_output>"
  [Vbus_required] -> MATLAB Function/10(Vdc_wanted)
  PV/1 -> Bus Selector2/1
  [curr_batt_command_3] -> Discrete PI Controller2/1(Error)  "Batt current command 3"
  From110/1 -> Discrete PI Controller3/1(Error)  "Batt current command 3"
  [Vbus_required] -> MATLAB Function1/3(Vbus_required)
  Bus Selector1/3 -> [Ibatt_command_pre]  "<current_command>"
  [Ifc_out] -> MATLAB Function/4(Ifc_out)
  [Vpv_conv] -> Vpv_conv/1
  Bus Selector1/2 -> [Ibatt]  "<Current (A)>"
  MATLAB Function1/3(V_batt_conv) -> [Vbatt_conv]
  [Ifc_boost] -> MATLAB Function/13(Ifc_boost)
  Bus Selector/2 -> [Ifc_boost_prev]  "<Ifc conv>"
  Bus Selector3/4 -> [Pload_real]  "<Pload real>"
  Discrete PI Controller3/1(Out) -> Sum9/2
  [Vbatt] -> MATLAB Function/1(Vbatt)
  Discrete PI Controller2/1(Out) -> Sum8/2
  Bus Selector1/5 -> [BATT_SOC]  "<SOC (%)>"
  Bus Selector1/4 -> [Ibatt_out]  "<Ibatt_output>"
  [Ipv_boost] -> Ipv_conv/1
  Bus Selector3/2 -> [Vbus_required]  "<Vbus required>"
  Bus Selector3/1 -> [Vbus_real]  "<Vbus real>"
  Bus Selector2/2 -> [Ipv_boost_prev]  "<PV current demand>"
  FC/1 -> Bus Selector/1
  Bus Selector/4 -> [Ifc_out]  "<Ifc out>"
  From26/1 -> Sum1/1  "Batt current command 1"
  [Pload_real] -> MATLAB Function/11(Pout)
  MATLAB Function1/2(current_command) -> [I_batt_charge]
  [Ibatt_out] -> MATLAB Function/3(Ibatt_out)
  SC/1 -> [SC_SOC]
  [Ipv] -> MATLAB Function/6(Ipv)
  Bus Selector2/1 -> [Vpv]  "<V_PV>"
  [Pload] -> MATLAB Function1/2(Pload)
  MATLAB Function/1(Ibatt_1) -> [curr_batt_command_1]
  Constant4/1 -> MATLAB Function/12(IO_batt_conv_value)
  MATLAB Function/2(Ibatt_2) -> [curr_batt_command_2]
  [IO_fc_boost] -> I/O fc conv/1
  [Ibatt] -> MATLAB Function/2(Ibatt)
  From108/1 -> Discrete PI Controller1/1(Error)  "Batt current command 1"
  [IO_pv_boost] -> I/O pv conv/1
  Bus Selector2/3 -> [Ipv]  "<I_PV>"
  [Vfc] -> MATLAB Function/14(Vfc)
  MATLAB Function/3(Ibatt_3) -> [curr_batt_command_3]
  From25/1 -> Sum1/2  "Batt current command 3"
  BATT/1 -> Bus Selector1/1
  [Ifc_boost] -> Ifc_conv/1
  [Vfc_conv] -> Vfc_conv/1
  Sum2/1 -> MATLAB Function1/1(current_comm)  "Batt current command"
  Bus Selector/1 -> [Vfc]  "<Vfc>"
  [Vpv] -> MATLAB Function/5(Vpv)
  [Vbus_real] -> MATLAB Function/9(Vdc)
  Bus Selector1/1 -> [Vbatt]  "<Voltage (V)>"
  Sum9/1 -> Sum8/1
  [Converter] -> batt converter mode/1
  MATLAB Function1/1(conv) -> [Converter]
  [I_batt_charge] -> Ibatt_conv/1
  Discrete PI Controller1/1(Out) -> Sum9/1
  Constant/1 -> PV - FC - control/14(IO_pv_conv_value)
  From40/1 -> PV - FC - control/10(SOC)
  PV - FC - control/7(Control_pv) -> Goto38/1
  From11/1 -> PV - FC - control/5(Vbatt)
  From41/1 -> PV - FC - control/8(Pload)
  PV - FC - control/5(Vpv_conv) -> Goto36/1
  Clock3/1 -> Zero-Order Hold/1  "time"
  From59/1 -> PV - FC - control/12(Vdc_real)
  From12/1 -> PV - FC - control/13(Pout_real)
  Constant10/1 -> PV - FC - control/16(Control_pv_choose_var)
  PV - FC - control/1(Ifc) -> Goto33/1
  From42/1 -> PV - FC - control/7(Vpv)
  PV - FC - control/3(IO_fc_conv) -> Goto35/1
  Zero-Order Hold/1 -> PV - FC - control/1(Time)  "time"
  From51/1 -> PV - FC - control/11(Ipvout)
  PV - FC - control/2(Vfc_conv) -> Goto34/1
  PV - FC - control/6(IO_pv_conv) -> Goto37/1
  From21/1 -> PV - FC - control/2(Vdc_command)
  PV - FC - control/4(Ipv) -> Goto6/1  "PV current demand"
  From44/1 -> PV - FC - control/4(Ifc_in)
  From73/1 -> PV - FC - control/6(Ibatt_in)
  Constant9/1 -> PV - FC - control/15(IO_fc_conv_value)
  From43/1 -> PV - FC - control/9(Ipv_in)
  From10/1 -> PV - FC - control/3(Vfc)
  Bus Selector/6 -> [limit]  "<limit>"
  Bus Selector/5 -> [E_act_d]  "<E_act_d>"
  Constant11/1 -> MATLAB Function2/10(sampleTime)
  Constant15/1 -> MATLAB Function2/11(Tmpc)
  Constant14/1 -> MATLAB Function2/12(IO_fc_conv)
  Constant13/1 -> MATLAB Function2/13(IO_pv_conv)
  Constant12/1 -> MATLAB Function2/14(Control_pv_choose_var)
  Clock2/1 -> Zero-Order Hold1/1
  MATLAB Function2/1(Vin) -> ?  "Vin_fcn_2"
  MATLAB Function2/3(Pin) -> ?  "Pin_fcn_2"
  MATLAB Function2/6(Pout) -> ?  "Pout_fcn_2"
  MATLAB Function2/5(Iout) -> ?  "Iout_fcn_2"
  MATLAB Function2/4(Vout) -> ?  "Vout_fcn_2"
  [Vfc_conv] -> Unit Delay/1
  [Ifc_boost] -> Unit Delay1/1
  [Ifc_out] -> MATLAB Function2/4(Ifc_out)
  [Vbus_real] -> MATLAB Function2/3(Vdc)
  [Ifc] -> MATLAB Function2/2("Iin ")
  [Vfc] -> MATLAB Function2/1("Vin ")
  [limit] -> MATLAB Function2/9(old_lim)
  [E_act_d] -> MATLAB Function2/8(old_E_act_d)
  MATLAB Function2/2(Iin) -> ?  "Iin_fcn_2"
  [Pload] -> MATLAB Function2/15(Pload)
  [BATT_SOC] -> MATLAB Function2/16(SOC)
  [Vbus_required] -> MATLAB Function2/18(Vdc_command)
  MATLAB Function2/7(Ifc_boost) -> [Ifc_boost]
  MATLAB Function2/8(Vfc_conv) -> [Vfc_conv]
  MATLAB Function2/9(IO_fc) -> [IO_fc_boost]
  MATLAB Function2/10(Ipv) -> [Ipv_boost]  "PV current demand"
  MATLAB Function2/11(Vpv_conv) -> [Vpv_conv]
  MATLAB Function2/12(IO_pv) -> [IO_pv_boost]
  MATLAB Function2/13(Control_pv) -> [Control_pv]
  Unit Delay/1 -> MATLAB Function2/5(Vdc_ref)
  Unit Delay1/1 -> MATLAB Function2/6(ILmax)
  Zero-Order Hold1/1 -> MATLAB Function2/7(time_data)
  [Ipv_out] -> MATLAB Function2/19(Ipv_out)
  [Pload_real] -> MATLAB Function2/20(Pout_real)
